simulink model "DC_SE_motor_control_sim"  (R2022b)
settings: Solver=VariableStepAuto  StartTime=0.0  StopTime=800  RelTol=1e-3
values from neighbouring files (symbols this model uses):
  B = Pfr/omega_n^2    (= 0.978238792649)    [DC_SE_motor_control.m]
  C1 = Vmax/omega_n    (= 0.0531210191083)    [DC_SE_motor_control.m]
  C3 = omega_n/60    (= 5.23333333333)    [DC_SE_motor_control.m]
  En = eta*Vn    (= 540)    [DC_SE_motor_control.m]
  Ie_n = 1    [DC_SE_motor_control.m]
  J = M*Vmax^2/omega_n^2    (= 73.3679094487)    [DC_SE_motor_control.m]
  K = Tn/(In*Ie_n)    (= 1.71974522293)    [DC_SE_motor_control.m]
  ki_curr = wia*Ra    (= 16.7961922659)    [DC_SE_motor_control.m]
  ki_ecc = wie*Re    (= 2400)    [DC_SE_motor_control.m]
  ki_speed = ws*B    (= 0.978238792649)    [DC_SE_motor_control.m]
  kp_curr = wia*La    (= 0.167961922659)    [DC_SE_motor_control.m]
  kp_ecc = wie*Le    (= 2400)    [DC_SE_motor_control.m]
  kp_speed = ws*J    (= 73.3679094487)    [DC_SE_motor_control.m]
  La = Ra*tau_a    (= 0.000839809613294)    [DC_SE_motor_control.m]
  Le = Re*tau_e    (= 120)    [DC_SE_motor_control.m]
  M = 10*1000+200*80    (= 26000)    [DC_SE_motor_control.m]
  omega_n = 314    [DC_SE_motor_control.m]
  Ra = (1-eta)*Vn/In    (= 0.0839809613294)    [DC_SE_motor_control.m]
  Re = Ve_n/Ie_n    (= 120)    [DC_SE_motor_control.m]
  Tn = Pn/omega_n    (= 1228.66792357)    [DC_SE_motor_control.m]
  Ve_n = 120    [DC_SE_motor_control.m]
  Vn = 600    [DC_SE_motor_control.m]
undefined symbols (not defined in the file or in its folder): sigbuilder_block
libraries: slpidlib x3
settings Model: Creator=anton  LastModifiedBy=anton

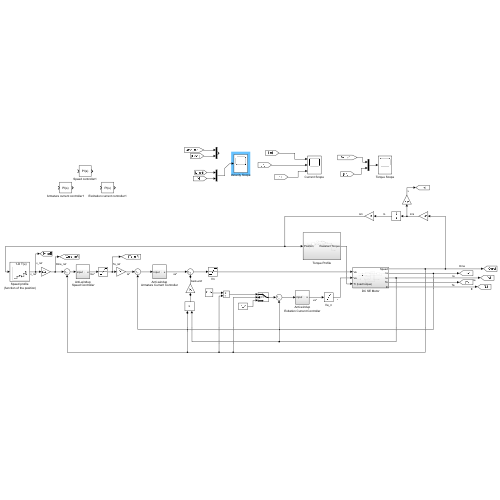
[thumbnail: Simulink's stored preview of the top-level diagram]
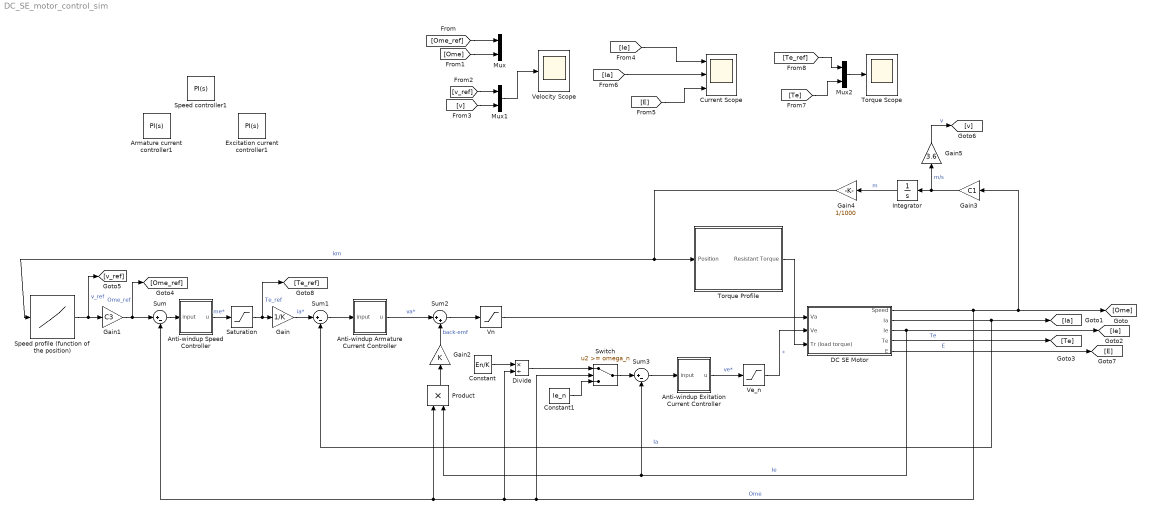
== system DC_SE_motor_control_sim ==
  Anti-windup Speed Controller : Subsystem
  Anti-windup Armature Current Controller : Subsystem
  Anti-windup Exitation Current Controller : Subsystem
  Armature current controller1 : slpidlib/PID Controller  Controller=PI  Form=Parallel  TimeDomain=Continuous-time  UseExternalTs=off  SampleTime=-1  IntegratorMethod=Forward Euler  FilterMethod=Forward Euler  ControllerParametersSource=internal  P=kp_curr  I=ki_curr  UseKiTs=off  D=0  N=100  UseFilter=on  TunerSelectOption=Transfer Function Based (PID Tuner App)  InitialConditionSource=internal  InitialConditionForIntegrator=0  InitialConditionForFilter=0  DifferentiatorICPrevScaledInput=0  ExternalReset=none  TrackingMode=off  Kt=1  LimitOutput=off  SatLimitsSource=internal  UpperSaturationLimit=inf  LowerSaturationLimit=-inf  LinearizeAsGain=on  AntiWindupMode=none  Kb=1  LimitIntegrator=off  UpperIntegratorSaturationLimit=inf  LowerIntegratorSaturationLimit=-inf  POutMin=[]  POutMax=[]  IOutMin=[]  IOutMax=[]  DOutMin=[]  DOutMax=[]  NOutMin=[]  NOutMax=[]  SumOutMin=[]  SumOutMax=[]  SaturationOutMin=[]  SaturationOutMax=[]  PParamMin=[]  PParamMax=[]  IParamMin=[]  IParamMax=[]  DParamMin=[]  DParamMax=[]  NParamMin=[]  NParamMax=[]  KbParamMin=[]  KbParamMax=[]  KtParamMin=[]  KtParamMax=[]  KbOutMin=[]  KbOutMax=[]  KtOutMin=[]  KtOutMax=[]  IntegratorOutMin=[]  IntegratorOutMax=[]  FilterOutMin=[]  FilterOutMax=[]  SumI1OutMin=[]  SumI1OutMax=[]  SumI2OutMin=[]  SumI2OutMax=[]  SumI3OutMin=[]  SumI3OutMax=[]  SumI4OutMin=[]  SumI4OutMax=[]  SumDOutMin=[]  SumDOutMax=[]  DifferentiatorOutMin=[]  DifferentiatorOutMax=[]  FilterDiffOutCoefMin=[]  FilterDiffOutCoefMax=[]  ReciprocalOutMin=[]  ReciprocalOutMax=[]  SumDenOutMin=[]  SumDenOutMax=[]  SumNumOutMin=[]  SumNumOutMax=[]  DivideOutMin=[]  DivideOutMax=[]  UdiffTsProdOutMin=[]  UdiffTsProdOutMax=[]  NTsProdOutMin=[]  NTsProdOutMax=[]  UintegralTsProdOutMin=[]  UintegralTsProdOutMax=[]  UngainTsProdOutMin=[]  UngainTsProdOutMax=[]  ClampingZeroOutDataTypeStr=Inherit: Inherit via back propagation  ClampingZeroOutMin=[]  ClampingZeroOutMax=[]  FilterDenConstantOutDataTypeStr=Inherit: Inherit via back propagation  FilterDenConstantOutMin=[]  FilterDenConstantOutMax=[]  PCopyOutDataTypeStr=Inherit: Inherit via back propagation  PCopyOutMin=[]  PCopyOutMax=[]  NCopyOutDataTypeStr=Inherit: Inherit via back propagation  NCopyOutMin=[]  NCopyOutMax=[]  IntegratorContinuousStateAttributes=''  IntegratorStateMustResolveToSignalObject=off  IntegratorRTWStateStorageClass=Auto  FilterContinuousStateAttributes=''  FilterStateMustResolveToSignalObject=off  FilterRTWStateStorageClass=Auto  ParallelPVariant=InternalParameters  IdealPVariant=Disabled  IVariant=InternalParameters  DVariant=Disabled  IntegratorVariant=Continuous  SatVariant=Disabled  AWVariant=Passthrough  PCopyVariant=Disabled  TRVariant=Disabled  FdbkBlocksVariant=Forward  IdealPFdbkVariant=Disabled  SatFdbkVariant=Disabled  DerivativeFilterVariant=Disabled  NVariant=Disabled  NCopyVariant=Disabled_SignalSpec  FilterICVariant=Disabled  IntegratorICVariant=InternalICs  ExternalResetVariant=Disabled  TRSumVariant=Passthrough  SumFdbkVariant=Disabled  SumVariant=Sum_PI  TsampFilterVariant=InternalTs  TsampNgainVariant=Passthrough  TsampIntegralVariant=Passthrough  ExternalSaturationOutDataTypeStr=Inherit: Same as second input
  Constant : Constant  Value=En/K
  Constant1 : Constant  Value=Ie_n
  Current Scope : Scope  NumInputPorts=3
  DC SE Motor : Subsystem
  Divide : Product  Inputs=*/
  Excitation current controller1 : slpidlib/PID Controller  Controller=PI  Form=Parallel  TimeDomain=Continuous-time  UseExternalTs=off  SampleTime=-1  IntegratorMethod=Forward Euler  FilterMethod=Forward Euler  ControllerParametersSource=internal  P=kp_ecc  I=ki_ecc  UseKiTs=off  D=0  N=100  UseFilter=on  TunerSelectOption=Transfer Function Based (PID Tuner App)  InitialConditionSource=internal  InitialConditionForIntegrator=0  InitialConditionForFilter=0  DifferentiatorICPrevScaledInput=0  ExternalReset=none  TrackingMode=off  Kt=1  LimitOutput=off  SatLimitsSource=internal  UpperSaturationLimit=inf  LowerSaturationLimit=-inf  LinearizeAsGain=on  AntiWindupMode=none  Kb=1  LimitIntegrator=off  UpperIntegratorSaturationLimit=inf  LowerIntegratorSaturationLimit=-inf  POutMin=[]  POutMax=[]  IOutMin=[]  IOutMax=[]  DOutMin=[]  DOutMax=[]  NOutMin=[]  NOutMax=[]  SumOutMin=[]  SumOutMax=[]  SaturationOutMin=[]  SaturationOutMax=[]  PParamMin=[]  PParamMax=[]  IParamMin=[]  IParamMax=[]  DParamMin=[]  DParamMax=[]  NParamMin=[]  NParamMax=[]  KbParamMin=[]  KbParamMax=[]  KtParamMin=[]  KtParamMax=[]  KbOutMin=[]  KbOutMax=[]  KtOutMin=[]  KtOutMax=[]  IntegratorOutMin=[]  IntegratorOutMax=[]  FilterOutMin=[]  FilterOutMax=[]  SumI1OutMin=[]  SumI1OutMax=[]  SumI2OutMin=[]  SumI2OutMax=[]  SumI3OutMin=[]  SumI3OutMax=[]  SumI4OutMin=[]  SumI4OutMax=[]  SumDOutMin=[]  SumDOutMax=[]  DifferentiatorOutMin=[]  DifferentiatorOutMax=[]  FilterDiffOutCoefMin=[]  FilterDiffOutCoefMax=[]  ReciprocalOutMin=[]  ReciprocalOutMax=[]  SumDenOutMin=[]  SumDenOutMax=[]  SumNumOutMin=[]  SumNumOutMax=[]  DivideOutMin=[]  DivideOutMax=[]  UdiffTsProdOutMin=[]  UdiffTsProdOutMax=[]  NTsProdOutMin=[]  NTsProdOutMax=[]  UintegralTsProdOutMin=[]  UintegralTsProdOutMax=[]  UngainTsProdOutMin=[]  UngainTsProdOutMax=[]  ClampingZeroOutDataTypeStr=Inherit: Inherit via back propagation  ClampingZeroOutMin=[]  ClampingZeroOutMax=[]  FilterDenConstantOutDataTypeStr=Inherit: Inherit via back propagation  FilterDenConstantOutMin=[]  FilterDenConstantOutMax=[]  PCopyOutDataTypeStr=Inherit: Inherit via back propagation  PCopyOutMin=[]  PCopyOutMax=[]  NCopyOutDataTypeStr=Inherit: Inherit via back propagation  NCopyOutMin=[]  NCopyOutMax=[]  IntegratorContinuousStateAttributes=''  IntegratorStateMustResolveToSignalObject=off  IntegratorRTWStateStorageClass=Auto  FilterContinuousStateAttributes=''  FilterStateMustResolveToSignalObject=off  FilterRTWStateStorageClass=Auto  ParallelPVariant=InternalParameters  IdealPVariant=Disabled  IVariant=InternalParameters  DVariant=Disabled  IntegratorVariant=Continuous  SatVariant=Disabled  AWVariant=Passthrough  PCopyVariant=Disabled  TRVariant=Disabled  FdbkBlocksVariant=Forward  IdealPFdbkVariant=Disabled  SatFdbkVariant=Disabled  DerivativeFilterVariant=Disabled  NVariant=Disabled  NCopyVariant=Disabled_SignalSpec  FilterICVariant=Disabled  IntegratorICVariant=InternalICs  ExternalResetVariant=Disabled  TRSumVariant=Passthrough  SumFdbkVariant=Disabled  SumVariant=Sum_PI  TsampFilterVariant=InternalTs  TsampNgainVariant=Passthrough  TsampIntegralVariant=Passthrough  ExternalSaturationOutDataTypeStr=Inherit: Same as second input
  Gain : Gain  Gain=1/K
  Gain1 : Gain  Gain=C3
  Gain2 : Gain  Gain=K
  Gain3 : Gain  Gain=C1
  Gain4 : Gain  Gain=1/1000
  Gain5 : Gain  Gain=3.6
  Integrator : Integrator
  Mux : Mux  Inputs=2
  Mux1 : Mux  Inputs=2
  Mux2 : Mux  Inputs=2
  Product : Product
  Saturation : Saturate  UpperLimit=Tn  LowerLimit=-Tn
  Speed controller1 : slpidlib/PID Controller  Controller=PI  Form=Parallel  TimeDomain=Continuous-time  UseExternalTs=off  SampleTime=-1  IntegratorMethod=Forward Euler  FilterMethod=Forward Euler  ControllerParametersSource=internal  P=kp_speed  I=ki_speed  UseKiTs=off  D=0  N=100  UseFilter=on  TunerSelectOption=Transfer Function Based (PID Tuner App)  InitialConditionSource=internal  InitialConditionForIntegrator=0  InitialConditionForFilter=0  DifferentiatorICPrevScaledInput=0  ExternalReset=none  TrackingMode=off  Kt=1  LimitOutput=off  SatLimitsSource=internal  UpperSaturationLimit=inf  LowerSaturationLimit=-inf  LinearizeAsGain=on  AntiWindupMode=none  Kb=1  LimitIntegrator=off  UpperIntegratorSaturationLimit=inf  LowerIntegratorSaturationLimit=-inf  POutMin=[]  POutMax=[]  IOutMin=[]  IOutMax=[]  DOutMin=[]  DOutMax=[]  NOutMin=[]  NOutMax=[]  SumOutMin=[]  SumOutMax=[]  SaturationOutMin=[]  SaturationOutMax=[]  PParamMin=[]  PParamMax=[]  IParamMin=[]  IParamMax=[]  DParamMin=[]  DParamMax=[]  NParamMin=[]  NParamMax=[]  KbParamMin=[]  KbParamMax=[]  KtParamMin=[]  KtParamMax=[]  KbOutMin=[]  KbOutMax=[]  KtOutMin=[]  KtOutMax=[]  IntegratorOutMin=[]  IntegratorOutMax=[]  FilterOutMin=[]  FilterOutMax=[]  SumI1OutMin=[]  SumI1OutMax=[]  SumI2OutMin=[]  SumI2OutMax=[]  SumI3OutMin=[]  SumI3OutMax=[]  SumI4OutMin=[]  SumI4OutMax=[]  SumDOutMin=[]  SumDOutMax=[]  DifferentiatorOutMin=[]  DifferentiatorOutMax=[]  FilterDiffOutCoefMin=[]  FilterDiffOutCoefMax=[]  ReciprocalOutMin=[]  ReciprocalOutMax=[]  SumDenOutMin=[]  SumDenOutMax=[]  SumNumOutMin=[]  SumNumOutMax=[]  DivideOutMin=[]  DivideOutMax=[]  UdiffTsProdOutMin=[]  UdiffTsProdOutMax=[]  NTsProdOutMin=[]  NTsProdOutMax=[]  UintegralTsProdOutMin=[]  UintegralTsProdOutMax=[]  UngainTsProdOutMin=[]  UngainTsProdOutMax=[]  ClampingZeroOutDataTypeStr=Inherit: Inherit via back propagation  ClampingZeroOutMin=[]  ClampingZeroOutMax=[]  FilterDenConstantOutDataTypeStr=Inherit: Inherit via back propagation  FilterDenConstantOutMin=[]  FilterDenConstantOutMax=[]  PCopyOutDataTypeStr=Inherit: Inherit via back propagation  PCopyOutMin=[]  PCopyOutMax=[]  NCopyOutDataTypeStr=Inherit: Inherit via back propagation  NCopyOutMin=[]  NCopyOutMax=[]  IntegratorContinuousStateAttributes=''  IntegratorStateMustResolveToSignalObject=off  IntegratorRTWStateStorageClass=Auto  FilterContinuousStateAttributes=''  FilterStateMustResolveToSignalObject=off  FilterRTWStateStorageClass=Auto  ParallelPVariant=InternalParameters  IdealPVariant=Disabled  IVariant=InternalParameters  DVariant=Disabled  IntegratorVariant=Continuous  SatVariant=Disabled  AWVariant=Passthrough  PCopyVariant=Disabled  TRVariant=Disabled  FdbkBlocksVariant=Forward  IdealPFdbkVariant=Disabled  SatFdbkVariant=Disabled  DerivativeFilterVariant=Disabled  NVariant=Disabled  NCopyVariant=Disabled_SignalSpec  FilterICVariant=Disabled  IntegratorICVariant=InternalICs  ExternalResetVariant=Disabled  TRSumVariant=Passthrough  SumFdbkVariant=Disabled  SumVariant=Sum_PI  TsampFilterVariant=InternalTs  TsampNgainVariant=Passthrough  TsampIntegralVariant=Passthrough  ExternalSaturationOutDataTypeStr=Inherit: Same as second input
  Speed profile (function of the position) : Lookup_n-D  NumberOfTableDimensions=1  BreakpointsForDimension1=[0 1 3 4 6 8 9 10]  Table=[35 60 60 75 60 60 35 0]  InterpMethod=Flat  InternalRulePriority=Speed  RndMeth=Simplest
  Sum : Sum  Inputs=|+-
  Sum1 : Sum  Inputs=|+-
  Sum2 : Sum  Inputs=|++
  Sum3 : Sum  Inputs=|+-
  Switch : Switch  Threshold=omega_n  SaturateOnIntegerOverflow=off  InputSameDT=off
  Torque Profile : Subsystem
  Torque Scope : Scope
  Ve_n : Saturate  UpperLimit=Ve_n  LowerLimit=-Ve_n
  Velocity Scope : Scope
  Vn : Saturate  UpperLimit=Vn  LowerLimit=-Vn
  wires:
  Gain1/1 -> [Ome_ref], Sum/1  "Ome_ref"
  DC SE Motor/1(Speed) -> Sum/2, Product/1, Divide/2, Switch/2, Gain3/1, [Ome]  "Ome"
  Torque Profile/1(Resistant Torque) -> DC SE Motor/3(Tr (load torque))
  Anti-windup Speed Controller/1(u) -> Saturation/1  "me*"
  Gain/1 -> Sum1/1  "ia*"
  DC SE Motor/2(Ia) -> Sum1/2, [Ia]  "Ia"
  Anti-windup Armature Current Controller/1(u) -> Sum2/1  "va*"
  Sum2/1 -> Vn/1
  Vn/1 -> DC SE Motor/1(Va)
  Gain2/1 -> Sum2/2  "back-emf"
  Product/1 -> Gain2/1
  Anti-windup Exitation Current Controller/1(u) -> Ve_n/1  "ve*"
  Ve_n/1 -> DC SE Motor/2(Ve)  "*"
  Sum3/1 -> Anti-windup Exitation Current Controller/1(input)
  DC SE Motor/3(Ie) -> Product/2, Sum3/2, [Ie]  "Ie"
  Switch/1 -> Sum3/1
  Divide/1 -> Switch/1
  Constant/1 -> Divide/1
  Constant1/1 -> Switch/3
  Gain3/1 -> Integrator/1, Gain5/1  "m/s"
  Integrator/1 -> Gain4/1  "m"
  Gain4/1 -> Speed profile (function of the position)/1, Torque Profile/1(Position)  "km"
  Speed profile (function of the position)/1 -> [v_ref], Gain1/1  "v_ref"
  DC SE Motor/4(Te) -> [Te]  "Te"
  Sum/1 -> Anti-windup Speed Controller/1(input)
  Sum1/1 -> Anti-windup Armature Current Controller/1(input)
  Saturation/1 -> [Te_ref], Gain/1  "Te_ref"
  [Ome] -> Mux/2
  [Ome_ref] -> Mux/1
  [v_ref] -> Mux1/1
  Gain5/1 -> [v]  "v"
  [v] -> Mux1/2
  Mux1/1 -> Velocity Scope/1
  DC SE Motor/5(E) -> [E]  "E"
  [Ie] -> Current Scope/1
  [E] -> Current Scope/3
  [Ia] -> Current Scope/2
  Mux2/1 -> Torque Scope/1
  [Te_ref] -> Mux2/1
  [Te] -> Mux2/2

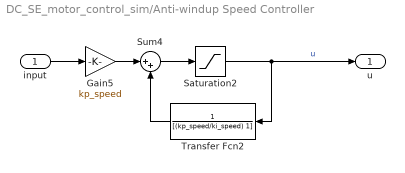
== system DC_SE_motor_control_sim/Anti-windup Speed Controller ==
  input : Inport
  Gain5 : Gain  Gain=kp_speed
  Saturation2 : Saturate  UpperLimit=Tn  LowerLimit=-Tn
  Sum4 : Sum  Inputs=|++
  Transfer Fcn2 : TransferFcn  Denominator=[(kp_speed/ki_speed) 1]
  u : Outport
  wires:
  input/1 -> Gain5/1
  Gain5/1 -> Sum4/1
  Transfer Fcn2/1 -> Sum4/2
  Saturation2/1 -> u/1, Transfer Fcn2/1  "u"
  Sum4/1 -> Saturation2/1

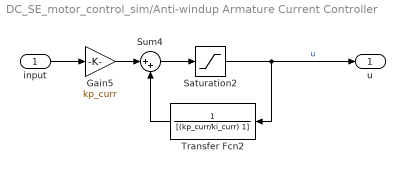
== system DC_SE_motor_control_sim/Anti-windup Armature Current Controller ==
  input : Inport
  Gain5 : Gain  Gain=kp_curr
  Saturation2 : Saturate  UpperLimit=Vn  LowerLimit=-Vn
  Sum4 : Sum  Inputs=|++
  Transfer Fcn2 : TransferFcn  Denominator=[(kp_curr/ki_curr) 1]
  u : Outport
  wires:
  input/1 -> Gain5/1
  Gain5/1 -> Sum4/1
  Transfer Fcn2/1 -> Sum4/2
  Saturation2/1 -> u/1, Transfer Fcn2/1  "u"
  Sum4/1 -> Saturation2/1

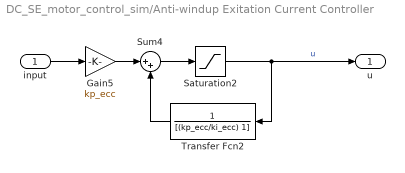
== system DC_SE_motor_control_sim/Anti-windup Exitation Current Controller ==
  input : Inport
  Gain5 : Gain  Gain=kp_ecc
  Saturation2 : Saturate  UpperLimit=Ve_n  LowerLimit=-Ve_n
  Sum4 : Sum  Inputs=|++
  Transfer Fcn2 : TransferFcn  Denominator=[(kp_ecc/ki_ecc) 1]
  u : Outport
  wires:
  input/1 -> Gain5/1
  Gain5/1 -> Sum4/1
  Transfer Fcn2/1 -> Sum4/2
  Saturation2/1 -> u/1, Transfer Fcn2/1  "u"
  Sum4/1 -> Saturation2/1

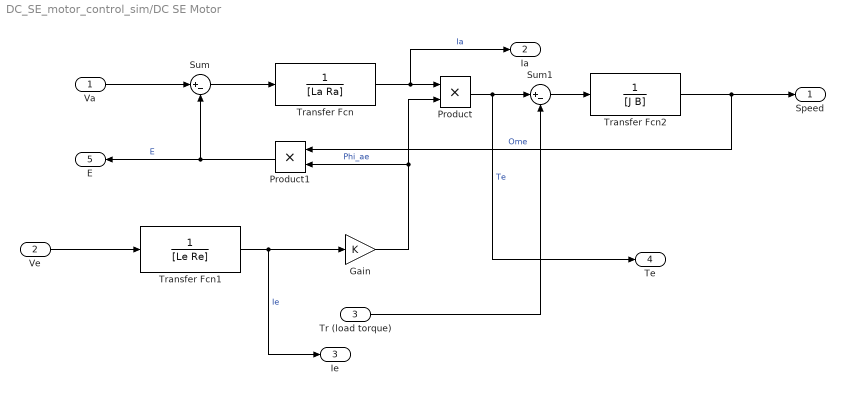
== system DC_SE_motor_control_sim/DC SE Motor ==
  Va : Inport
  Ve : Inport  Port=2
  Tr (load torque) : Inport  Port=3
  Gain : Gain  Gain=K
  Product : Product
  Product1 : Product
  Sum : Sum  Inputs=|+-
  Sum1 : Sum  Inputs=|+-
  Transfer Fcn : TransferFcn  Denominator=[La Ra]
  Transfer Fcn1 : TransferFcn  Denominator=[Le Re]
  Transfer Fcn2 : TransferFcn  Denominator=[J B]
  Speed : Outport
  Ia : Outport  Port=2
  Ie : Outport  Port=3
  Te : Outport  Port=4
  E : Outport  Port=5
  wires:
  Product1/1 -> E/1, Sum/2  "E"
  Va/1 -> Sum/1
  Sum/1 -> Transfer Fcn/1
  Transfer Fcn/1 -> Ia/1, Product/1  "Ia"
  Gain/1 -> Product1/2, Product/2  "Phi_ae"
  Ve/1 -> Transfer Fcn1/1
  Transfer Fcn2/1 -> Product1/1, Speed/1  "Ome"
  Transfer Fcn1/1 -> Ie/1, Gain/1  "Ie"
  Product/1 -> Te/1, Sum1/1  "Te"
  Tr (load torque)/1 -> Sum1/2
  Sum1/1 -> Transfer Fcn2/1

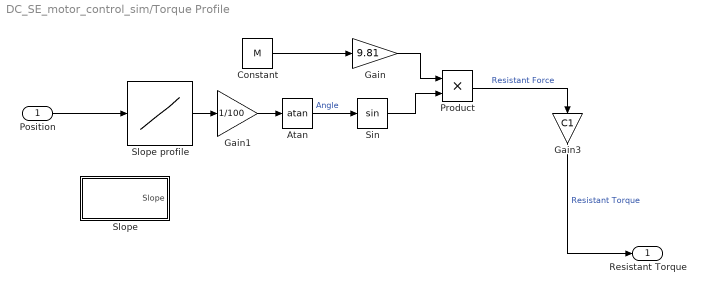
== system DC_SE_motor_control_sim/Torque Profile ==
  Position : Inport
  Atan : Trigonometry  Operator=atan
  Constant : Constant  Value=M
  Gain : Gain  Gain=9.81
  Gain1 : Gain  Gain=1/100
  Gain3 : Gain  Gain=C1
  Product : Product
  Sin : Trigonometry
  Slope : Subsystem  Tag=STV Subsys  LoadFcn=sigbuilder_block('load');  StartFcn=sigbuilder_block('start');  StopFcn=sigbuilder_block('stop');  ClipboardFcn=sigbuilder_block('clipboard');  mask(Sigbuilder block){tuvar=[0:10]}
      mask help: Simulink:masks:SigbuilderBlock_MD
      mask init:
      | if ~strcmp(get_param(bdroot(gcbh),'SimulationStatus'),'stopped') tuvar = sigbuilder_block('maskInit'); end
      settings: CopyFcn=sigbuilder_block('copy');  DeleteFcn=sigbuilder_block('delete');  ModelCloseFcn=sigbuilder_block('modelClose');  PreSaveFcn=sigbuilder_block('preSave');  PauseFcn=sigbuilder_block('pause');  ContinueFcn=sigbuilder_block('continue');  NameChangeFcn=sigbuilder_block('namechange');  OpenFcn=sigbuilder_block('open',[505.8 109.8 550.8 400.2 ]);  CloseFcn=sigbuilder_block('close');
      mask Display: plot(0, 0, 100, 100,[2, 2, 32, 32, 2], [68, 8, 8, 68, 68],[32, 2], [38, 38], [32, 19, 2],[53, 60, 44], [32, 17, 17, 2],[16, 16, 31, 31]);txt = getActiveGroup(gcbh);text(2, 100, txt,'verticalAlignment', 'top');
  Slope profile : Lookup_n-D  NumberOfTableDimensions=1  BreakpointsForDimension1=[0 1 3 4 6 8 9 10]  Table=[0 0 5 0 0 0 -5 0]  InterpMethod=Flat  InternalRulePriority=Speed  RndMeth=Simplest
  Resistant Torque : Outport
  wires:
  Sin/1 -> Product/2
  Gain3/1 -> Resistant Torque/1  "Resistant Torque"
  Product/1 -> Gain3/1  "Resistant Force"
  Gain/1 -> Product/1
  Constant/1 -> Gain/1
  Atan/1 -> Sin/1  "Angle"
  Position/1 -> Slope profile/1
  Slope profile/1 -> Gain1/1
  Gain1/1 -> Atan/1

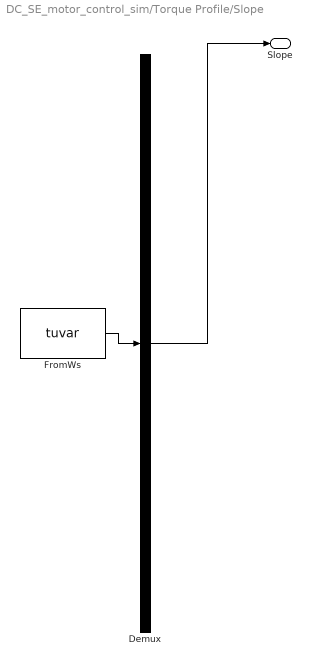
== system DC_SE_motor_control_sim/Torque Profile/Slope ==
  Demux : Demux  Tag=STV Demux  Outputs=1
      settings: DisplayOption=none
  FromWs : FromWorkspace  Tag=STV FromWs  VariableName=tuvar
      SigBuilderData=|
      | common.afterFinalStr = 'Extrapolate'
      | common.sampleTime = 0
      | dataSet.timeRange = [0 721.7143]
      | dataSet.name = 'Group 1'
      | sbobj.Groups.Name = 'Group 1'
      | sbobj.Groups.Signals.Name = 'Slope'
      | sbobj.Groups.Signals.XData = [0 102.8571 282.8571 282.8571 342.8571 342.8571 438.8571 558.8571 558.8571 618.8571 618.8571 721.7143]
      | sbobj.Groups.Signals.YData = [0 0 0 0.05 0.05 0 0 0 -0.05 -0.05 0 0]
      | sbobj.Groups.TimeRange = [0 721.7143]
  Slope : Outport  Tag=STV Outport
  wires:
  FromWs/1 -> Demux/1
  Demux/1 -> Slope/1
